simulink model "forward_speed_model_ulin_2"  (R2017b)
settings: Solver=ode45  StartTime=tstart  StopTime=tstop  RelTol=1e-3  EnableMultiTasking=on
values from neighbouring files (symbols this model uses):
  k = lsqcurvefit(F, k0, t, u,[600 0.2 0.09],[1150 0.6  0.13],OPT)    [analyse_dynamics_v3.m]    (also in analysis_dynamics.m = lsqcurvefit(F3,k0,t,u,lb,ub,options))
  tau_1 = n_c    [sim_forward_speed_mass_damp_model.m]    (also in sim_forward_speed_model_ulin.m)
  tsamp = 100    [analyse_dynamics_v3.m]    (also in analysis_dynamics.m; run.m = 10; run_task_1_8.m = 10)
settings Model: ExtModeAutoUpdateStatusClock=off  Creator=christh  LastModifiedBy=EllaLovise
settings DataIOCC: LimitDataPoints=on  SaveFormat=Array  SignalLoggingSaveFormat=ModelDataLogs
settings OptimizationCC: ExpressionDepthLimit=2147483647  InitFltsAndDblsToZero=on  LifeSpan=inf
settings DebuggingCC: UnderspecifiedInitializationDetection=Classic  MergeDetectMultiDrivingBlocksExec=none  SolverPrmCheckMsg=warning  FcnCallInpInsideContextMsg=warning  StateNameClashWarn=warning  SFUnexpectedBacktrackingDiag=warning  SFNoUnconditionalDefaultTransitionDiag=warning  SFExecutionAtInitializationDiag=none
settings HardwareCC: ProdBitPerPointer=32  ProdBitPerSizeT=32  ProdBitPerPtrDiffT=32  ProdLargestAtomicFloat=None  ProdIntDivRoundTo=Undefined  ProdEndianess=Unspecified  ProdWordSize=32  ProdHWDeviceType=32-bit Generic
settings ModelReferenceCC: PropagateSignalLabelsOutOfModel=off
settings CodeAppCC: StateflowObjectComments=on
settings GRTTargetCC: TargetLangStandard=C89/C90 (ANSI)  GeneratePreprocessorConditionals=Disable all  CombineOutputUpdateFcns=off  GRTInterface=on
settings ConfigComp: CovMetricSettings=dw  CovHtmlReporting=on  CovSaveCumulativeToWorkspaceVar=on  CovSaveSingleToWorkspaceVar=on  CovExternalEMLEnable=off

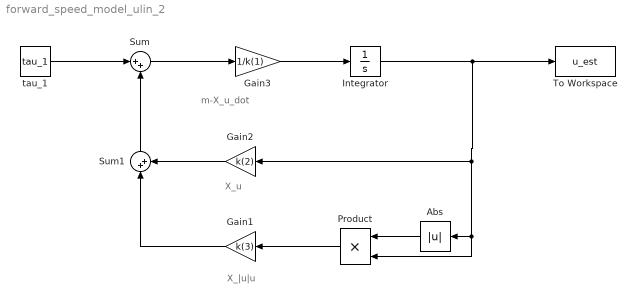
== system forward_speed_model_ulin_2 ==
  note: X_u
  note: X_|u|u
  note: m-X_u_dot
  Abs : Abs
  Gain1 : Gain  Gain=k(3)
  Gain2 : Gain  Gain=k(2)
  Gain3 : Gain  Gain=1/k(1)
  Integrator : Integrator
  Product : Product
  Sum : Sum  Inputs=|++
  Sum1 : Sum  Inputs=|++
  To Workspace : ToWorkspace  VariableName=u_est  SaveFormat=Timeseries  SampleTime=tsamp
  tau_1 : Constant  Value=tau_1
  wires:
  Gain2/1 -> Sum1/2
  Gain1/1 -> Sum1/1
  Sum1/1 -> Sum/2
  tau_1/1 -> Sum/1
  Sum/1 -> Gain3/1
  Product/1 -> Gain1/1
  Integrator/1 -> To Workspace/1, Product/2, Abs/1, Gain2/1
  Abs/1 -> Product/1
  Gain3/1 -> Integrator/1
